simulink subsystem "FCS_Fixed_Wing"  (R2025a)
settings: Solver=VariableStepAuto  StartTime=0.0  StopTime=10.0  RelTol=1e-3
settings Model: Creator=gurt1  LastModifiedBy=gurt1
settings RTWCC: GPUComputeCapability=3.5

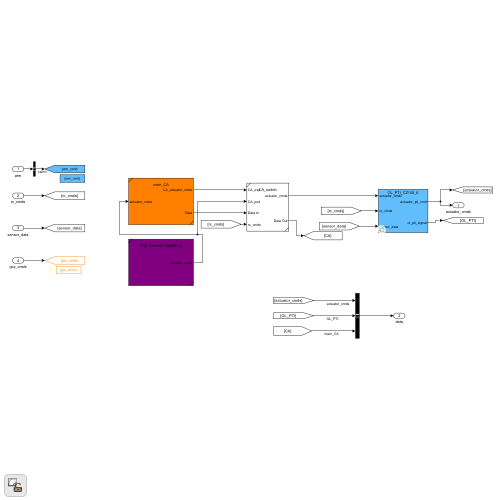
[thumbnail: Simulink's stored preview of the top-level diagram]
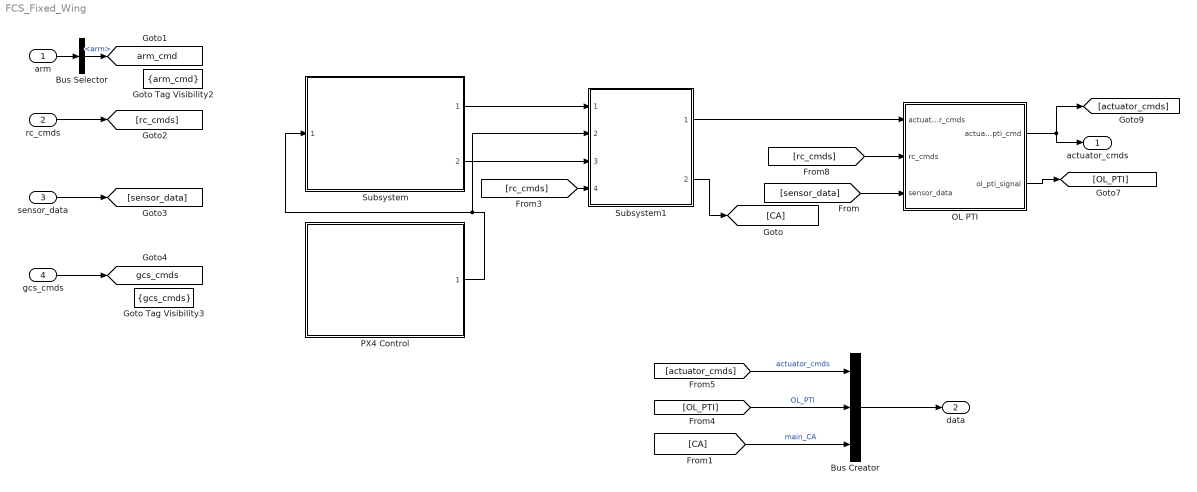
== system FCS_Fixed_Wing ==
  arm : Inport
  rc_cmds : Inport  Port=2
  sensor_data : Inport  Port=3
  gcs_cmds : Inport  Port=4
  Bus Creator : BusCreator  Inputs=3
  Bus Selector : BusSelector  OutputSignals=arm
  Goto Tag Visibility2 : GotoTagVisibility  GotoTag=arm_cmd
  Goto Tag Visibility3 : GotoTagVisibility  GotoTag=gcs_cmds
  OL PTI : Subsystem  Variant=on  EmptyChoice=on
  PX4 Control : Subsystem  ReferencedSubsystem=PX4_Control_FixedWing
  Subsystem : Subsystem  ReferencedSubsystem=main_CA
  Subsystem1 : Subsystem  ReferencedSubsystem=CA_switch
  actuator_cmds : Outport
  data : Outport  Port=2
  tag scope: arm_cmd=global, gcs_cmds=global
  wires:
  Bus Creator/1 -> data/1
  [actuator_cmds] -> Bus Creator/1  "actuator_cmds"
  [OL_PTI] -> Bus Creator/2  "OL_PTI"
  rc_cmds/1 -> [rc_cmds]
  sensor_data/1 -> [sensor_data]
  gcs_cmds/1 -> [gcs_cmds]
  Bus Selector/1 -> [arm_cmd]  "<arm>"
  arm/1 -> Bus Selector/1
  Subsystem1/1 -> OL PTI/1(actuator_cmds)
  [rc_cmds] -> OL PTI/2(rc_cmds)
  [sensor_data] -> OL PTI/3(sensor_data)
  OL PTI/1(actuator_pti_cmd) -> actuator_cmds/1, [actuator_cmds]
  OL PTI/2(ol_pti_signal) -> [OL_PTI]
  Subsystem/1 -> Subsystem1/1
  PX4 Control/1 -> Subsystem/1, Subsystem1/2
  [rc_cmds] -> Subsystem1/4
  Subsystem/2 -> Subsystem1/3
  Subsystem1/2 -> [CA]
  [CA] -> Bus Creator/3  "main_CA"

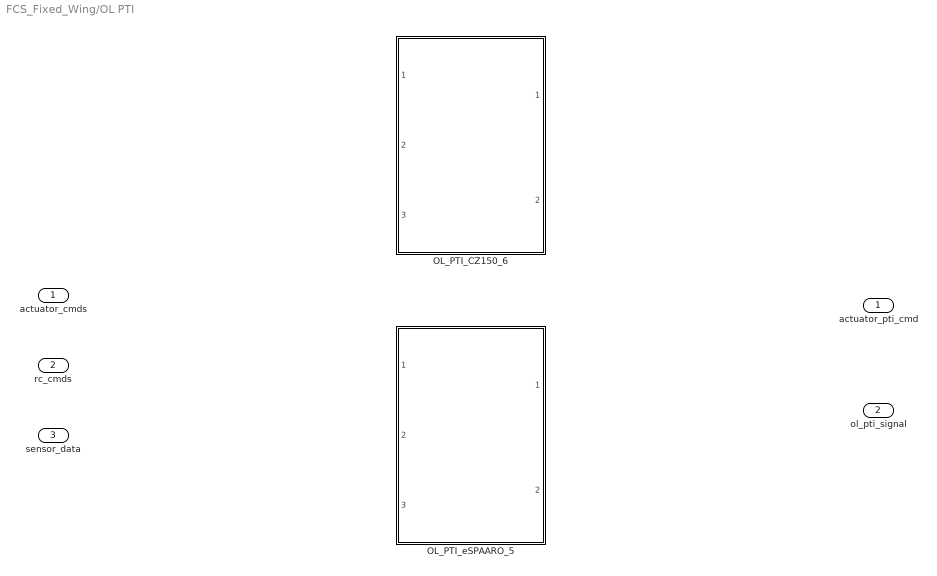
== system FCS_Fixed_Wing/OL PTI ==
  actuator_cmds : Inport
  rc_cmds : Inport  Port=2
  sensor_data : Inport  Port=3
  OL_PTI_CZ150_6 : Subsystem  VariantControl=FW_type == 1  ReferencedSubsystem=OL_PTI_CZ150_6
  OL_PTI_eSPAARO_5 : Subsystem  VariantControl=FW_type == 2  ReferencedSubsystem=OL_PTI_eSPAARO_5
  actuator_pti_cmd : Outport
  ol_pti_signal : Outport  Port=2
